simulink model "OptimizationCar"  (Simulink 8.8)
settings: Solver=FixedStepAuto  StartTime=0.0  StopTime=10.0  RelTol=1e-3
model workspace: external: MAT-File C:\Users\EMIdev1\Documents\GitHub\DRI001-MPS-2018.2.3-601-2\DRI006\DRIPSamples\CollisionWarningSystem\external\SlkModels\OptimizationCar.mat (data not in the file)
undefined symbols (not defined in the file or in its folder): detectionRange, driverReacionTime, frictionCoef, subjectPosition, subjectVelocity, targetPosition, targetVelocity
(part 1 of 2)
settings Model: Creator=EMIdev1  LastModifiedBy=EMIdev1
settings DataIOCC: LimitDataPoints=off  SaveFormat=Dataset  SignalLoggingSaveFormat=Dataset
settings OptimizationCC: LifeSpan=auto
settings DebuggingCC: UnderspecifiedInitializationDetection=Simplified  MergeDetectMultiDrivingBlocksExec=error  FcnCallInpInsideContextMsg=error  StateNameClashWarn=none  SFUnexpectedBacktrackingDiag=error  SFNoUnconditionalDefaultTransitionDiag=error  SFExecutionAtInitializationDiag=warning
settings HardwareCC: ProdLargestAtomicFloat=Float  ProdIntDivRoundTo=Zero  ProdEndianess=LittleEndian  ProdHWDeviceType=Intel->x86-32 (Windows32)
settings ModelReferenceCC: PropagateSignalLabelsOutOfModel=on
settings GRTTargetCC: TargetLangStandard=C99 (ISO)  GeneratePreprocessorConditionals=Use local settings  CombineOutputUpdateFcns=on  GRTInterface=off
settings ConfigComp: CovMetricSettings=dwe  CovHtmlReporting=off  CovSaveCumulativeToWorkspaceVar=off  CovSaveSingleToWorkspaceVar=off  CovExternalEMLEnable=on

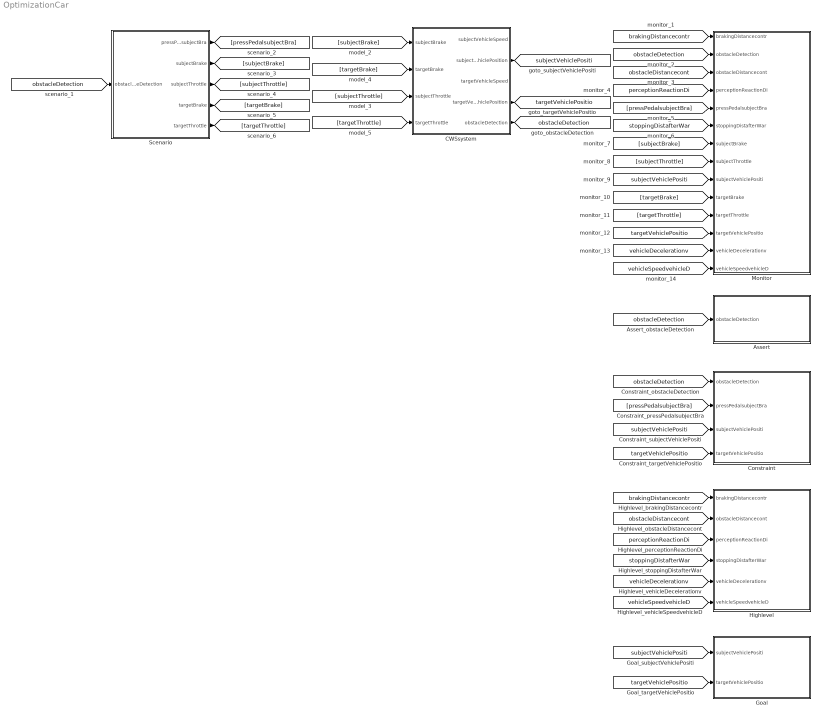
== system OptimizationCar ==
  Assert : Subsystem
  CWSsystem : Subsystem  LoadFcn=""
  Constraint : Subsystem
  Goal : Subsystem
  Highlevel : Subsystem
  Monitor : Subsystem
  Scenario : Subsystem
  tag scope: obstacleDetection=global, subjectVehiclePositi=global, targetVehiclePositio=global
  wires:
  [obstacleDetection] -> Scenario/1(obstacleDetection)
  Scenario/1(pressPedalsubjectBra) -> [pressPedalsubjectBra]
  Scenario/2(subjectBrake) -> [subjectBrake]
  [subjectBrake] -> CWSsystem/1(subjectBrake)
  Scenario/3(subjectThrottle) -> [subjectThrottle]
  [subjectThrottle] -> CWSsystem/3(subjectThrottle)
  Scenario/4(targetBrake) -> [targetBrake]
  [targetBrake] -> CWSsystem/2(targetBrake)
  Scenario/5(targetThrottle) -> [targetThrottle]
  [targetThrottle] -> CWSsystem/4(targetThrottle)
  [brakingDistancecontr] -> Monitor/1(brakingDistancecontr)
  [obstacleDetection] -> Monitor/2(obstacleDetection)
  [obstacleDistancecont] -> Monitor/3(obstacleDistancecont)
  [perceptionReactionDi] -> Monitor/4(perceptionReactionDi)
  [pressPedalsubjectBra] -> Monitor/5(pressPedalsubjectBra)
  [stoppingDistafterWar] -> Monitor/6(stoppingDistafterWar)
  [subjectBrake] -> Monitor/7(subjectBrake)
  [subjectThrottle] -> Monitor/8(subjectThrottle)
  [subjectVehiclePositi] -> Monitor/9(subjectVehiclePositi)
  [targetBrake] -> Monitor/10(targetBrake)
  [targetThrottle] -> Monitor/11(targetThrottle)
  [targetVehiclePositio] -> Monitor/12(targetVehiclePositio)
  [vehicleDecelerationv] -> Monitor/13(vehicleDecelerationv)
  [vehicleSpeedvehicleD] -> Monitor/14(vehicleSpeedvehicleD)
  [obstacleDetection] -> Assert/1(obstacleDetection)
  [obstacleDetection] -> Constraint/1(obstacleDetection)
  [pressPedalsubjectBra] -> Constraint/2(pressPedalsubjectBra)
  [subjectVehiclePositi] -> Constraint/3(subjectVehiclePositi)
  [targetVehiclePositio] -> Constraint/4(targetVehiclePositio)
  [brakingDistancecontr] -> Highlevel/1(brakingDistancecontr)
  [obstacleDistancecont] -> Highlevel/2(obstacleDistancecont)
  [perceptionReactionDi] -> Highlevel/3(perceptionReactionDi)
  [stoppingDistafterWar] -> Highlevel/4(stoppingDistafterWar)
  [vehicleDecelerationv] -> Highlevel/5(vehicleDecelerationv)
  [vehicleSpeedvehicleD] -> Highlevel/6(vehicleSpeedvehicleD)
  [subjectVehiclePositi] -> Goal/1(subjectVehiclePositi)
  [targetVehiclePositio] -> Goal/2(targetVehiclePositio)
  CWSsystem/5(obstacleDetection) -> [obstacleDetection]
  CWSsystem/2(subjectVehiclePosition) -> [subjectVehiclePositi]
  CWSsystem/4(targetVehiclePosition) -> [targetVehiclePositio]

== system OptimizationCar/Assert ==
  obstacleDetection : Inport
  Assert_1 : Subsystem
  simout_1 : ToFile  Filename=Assert_1.mat  MatrixName=Assert_1  SaveFormat=Timeseries
  wires:
  obstacleDetection/1 -> Assert_1/1(obstacleDetection)
  Assert_1/1(Assert_1) -> simout_1/1

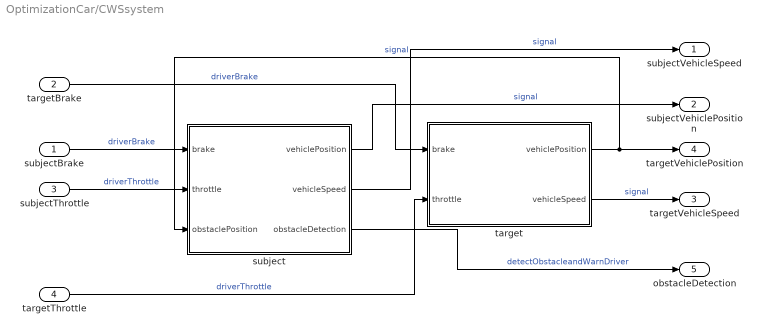
== system OptimizationCar/CWSsystem ==
  subjectBrake : Inport
      settings: AttributesFormatString=driverBrake
  targetBrake : Inport  Port=2
      settings: AttributesFormatString=driverBrake
  subjectThrottle : Inport  Port=3
      settings: AttributesFormatString=driverThrottle
  targetThrottle : Inport  Port=4
      settings: AttributesFormatString=driverThrottle
  subject : Subsystem  LoadFcn=""
  target : Subsystem  LoadFcn=""
  subjectVehicleSpeed : Outport
      settings: AttributesFormatString=signal
  subjectVehiclePosition : Outport  Port=2
      settings: AttributesFormatString=signal
  targetVehicleSpeed : Outport  Port=3
      settings: AttributesFormatString=signal
  targetVehiclePosition : Outport  Port=4
      settings: AttributesFormatString=signal
  obstacleDetection : Outport  Port=5
      settings: AttributesFormatString=detectObstacleandWarnDriver
  wires:
  subject/3(obstacleDetection) -> obstacleDetection/1  "detectObstacleandWarnDriver"
  target/2(vehicleSpeed) -> targetVehicleSpeed/1  "signal"
  subject/2(vehicleSpeed) -> subjectVehicleSpeed/1  "signal"
  subject/1(vehiclePosition) -> subjectVehiclePosition/1  "signal"
  targetThrottle/1 -> target/2(throttle)  "driverThrottle"
  subjectThrottle/1 -> subject/2(throttle)  "driverThrottle"
  targetBrake/1 -> target/1(brake)  "driverBrake"
  subjectBrake/1 -> subject/1(brake)  "driverBrake"
  target/1(vehiclePosition) -> targetVehiclePosition/1, subject/3(obstaclePosition)  "signal"

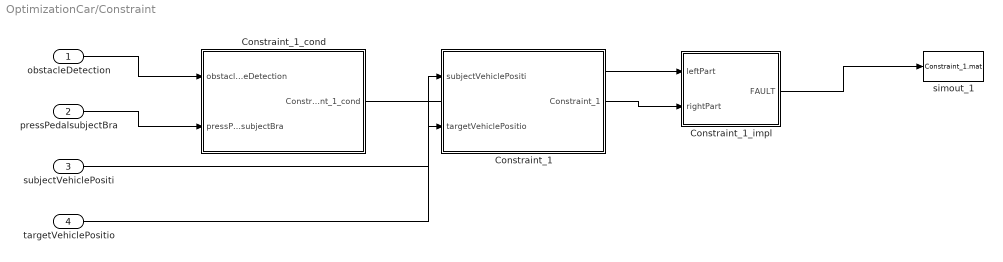
== system OptimizationCar/Constraint ==
  obstacleDetection : Inport
  pressPedalsubjectBra : Inport  Port=2
  subjectVehiclePositi : Inport  Port=3
  targetVehiclePositio : Inport  Port=4
  Constraint_1 : Subsystem
  Constraint_1_cond : Subsystem
  Constraint_1_impl : Subsystem  TreatAsAtomicUnit=on
  simout_1 : ToFile  Filename=Constraint_1.mat  MatrixName=Constraint_1  SaveFormat=Timeseries
  wires:
  obstacleDetection/1 -> Constraint_1_cond/1(obstacleDetection)
  pressPedalsubjectBra/1 -> Constraint_1_cond/2(pressPedalsubjectBra)
  Constraint_1_cond/1(Constraint_1_cond) -> Constraint_1_impl/1(leftPart)
  subjectVehiclePositi/1 -> Constraint_1/1(subjectVehiclePositi)
  targetVehiclePositio/1 -> Constraint_1/2(targetVehiclePositio)
  Constraint_1/1(Constraint_1) -> Constraint_1_impl/2(rightPart)
  Constraint_1_impl/1(FAULT) -> simout_1/1

== system OptimizationCar/Goal ==
  subjectVehiclePositi : Inport
  targetVehiclePositio : Inport  Port=2
  Goal_1 : Subsystem
  simout_1 : ToFile  Filename=Goal_1.mat  MatrixName=Goal_1  SaveFormat=Timeseries
  wires:
  subjectVehiclePositi/1 -> Goal_1/1(subjectVehiclePositi)
  targetVehiclePositio/1 -> Goal_1/2(targetVehiclePositio)
  Goal_1/1(Goal_1) -> simout_1/1

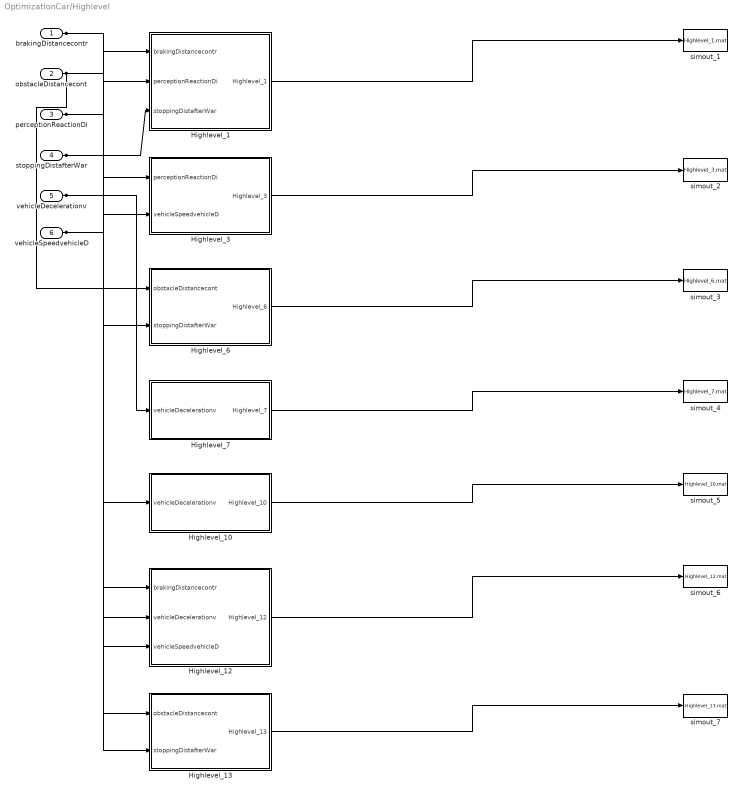
== system OptimizationCar/Highlevel ==
  brakingDistancecontr : Inport
  obstacleDistancecont : Inport  Port=2
  perceptionReactionDi : Inport  Port=3
  stoppingDistafterWar : Inport  Port=4
  vehicleDecelerationv : Inport  Port=5
  vehicleSpeedvehicleD : Inport  Port=6
  Highlevel_1 : Subsystem
  Highlevel_10 : Subsystem
  Highlevel_12 : Subsystem
  Highlevel_13 : Subsystem
  Highlevel_3 : Subsystem
  Highlevel_6 : Subsystem
  Highlevel_7 : Subsystem
  simout_1 : ToFile  Filename=Highlevel_1.mat  MatrixName=Highlevel_1  SaveFormat=Timeseries
  simout_2 : ToFile  Filename=Highlevel_3.mat  MatrixName=Highlevel_3  SaveFormat=Timeseries
  simout_3 : ToFile  Filename=Highlevel_6.mat  MatrixName=Highlevel_6  SaveFormat=Timeseries
  simout_4 : ToFile  Filename=Highlevel_7.mat  MatrixName=Highlevel_7  SaveFormat=Timeseries
  simout_5 : ToFile  Filename=Highlevel_10.mat  MatrixName=Highlevel_10  SaveFormat=Timeseries
  simout_6 : ToFile  Filename=Highlevel_12.mat  MatrixName=Highlevel_12  SaveFormat=Timeseries
  simout_7 : ToFile  Filename=Highlevel_13.mat  MatrixName=Highlevel_13  SaveFormat=Timeseries
  wires:
  brakingDistancecontr/1 -> Highlevel_1/1(brakingDistancecontr), Highlevel_12/1(brakingDistancecontr)
  perceptionReactionDi/1 -> Highlevel_1/2(perceptionReactionDi), Highlevel_3/1(perceptionReactionDi)
  stoppingDistafterWar/1 -> Highlevel_1/3(stoppingDistafterWar), Highlevel_6/2(stoppingDistafterWar), Highlevel_13/2(stoppingDistafterWar)
  Highlevel_1/1(Highlevel_1) -> simout_1/1
  vehicleSpeedvehicleD/1 -> Highlevel_3/2(vehicleSpeedvehicleD), Highlevel_12/3(vehicleSpeedvehicleD)
  Highlevel_3/1(Highlevel_3) -> simout_2/1
  obstacleDistancecont/1 -> Highlevel_6/1(obstacleDistancecont), Highlevel_13/1(obstacleDistancecont)
  Highlevel_6/1(Highlevel_6) -> simout_3/1
  vehicleDecelerationv/1 -> Highlevel_7/1(vehicleDecelerationv), Highlevel_10/1(vehicleDecelerationv), Highlevel_12/2(vehicleDecelerationv)
  Highlevel_7/1(Highlevel_7) -> simout_4/1
  Highlevel_10/1(Highlevel_10) -> simout_5/1
  Highlevel_12/1(Highlevel_12) -> simout_6/1
  Highlevel_13/1(Highlevel_13) -> simout_7/1

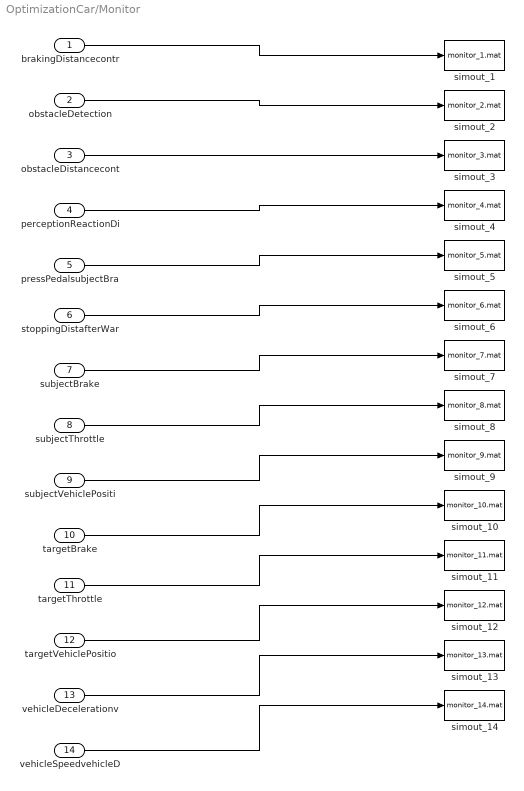
== system OptimizationCar/Monitor ==
  brakingDistancecontr : Inport
  obstacleDetection : Inport  Port=2
  obstacleDistancecont : Inport  Port=3
  perceptionReactionDi : Inport  Port=4
  pressPedalsubjectBra : Inport  Port=5
  stoppingDistafterWar : Inport  Port=6
  subjectBrake : Inport  Port=7
  subjectThrottle : Inport  Port=8
  subjectVehiclePositi : Inport  Port=9
  targetBrake : Inport  Port=10
  targetThrottle : Inport  Port=11
  targetVehiclePositio : Inport  Port=12
  vehicleDecelerationv : Inport  Port=13
  vehicleSpeedvehicleD : Inport  Port=14
  simout_1 : ToFile  Filename=monitor_1.mat  MatrixName=brakingDistancecontr  SaveFormat=Timeseries
  simout_10 : ToFile  Filename=monitor_10.mat  MatrixName=targetBrake  SaveFormat=Timeseries
  simout_11 : ToFile  Filename=monitor_11.mat  MatrixName=targetThrottle  SaveFormat=Timeseries
  simout_12 : ToFile  Filename=monitor_12.mat  MatrixName=targetVehiclePositio  SaveFormat=Timeseries
  simout_13 : ToFile  Filename=monitor_13.mat  MatrixName=vehicleDecelerationv  SaveFormat=Timeseries
  simout_14 : ToFile  Filename=monitor_14.mat  MatrixName=vehicleSpeedvehicleD  SaveFormat=Timeseries
  simout_2 : ToFile  Filename=monitor_2.mat  MatrixName=obstacleDetection  SaveFormat=Timeseries
  simout_3 : ToFile  Filename=monitor_3.mat  MatrixName=obstacleDistancecont  SaveFormat=Timeseries
  simout_4 : ToFile  Filename=monitor_4.mat  MatrixName=perceptionReactionDi  SaveFormat=Timeseries
  simout_5 : ToFile  Filename=monitor_5.mat  MatrixName=pressPedalsubjectBra  SaveFormat=Timeseries
  simout_6 : ToFile  Filename=monitor_6.mat  MatrixName=stoppingDistafterWar  SaveFormat=Timeseries
  simout_7 : ToFile  Filename=monitor_7.mat  MatrixName=subjectBrake  SaveFormat=Timeseries
  simout_8 : ToFile  Filename=monitor_8.mat  MatrixName=subjectThrottle  SaveFormat=Timeseries
  simout_9 : ToFile  Filename=monitor_9.mat  MatrixName=subjectVehiclePositi  SaveFormat=Timeseries
  wires:
  brakingDistancecontr/1 -> simout_1/1
  obstacleDetection/1 -> simout_2/1
  obstacleDistancecont/1 -> simout_3/1
  perceptionReactionDi/1 -> simout_4/1
  pressPedalsubjectBra/1 -> simout_5/1
  stoppingDistafterWar/1 -> simout_6/1
  subjectBrake/1 -> simout_7/1
  subjectThrottle/1 -> simout_8/1
  subjectVehiclePositi/1 -> simout_9/1
  targetBrake/1 -> simout_10/1
  targetThrottle/1 -> simout_11/1
  targetVehiclePositio/1 -> simout_12/1
  vehicleDecelerationv/1 -> simout_13/1
  vehicleSpeedvehicleD/1 -> simout_14/1

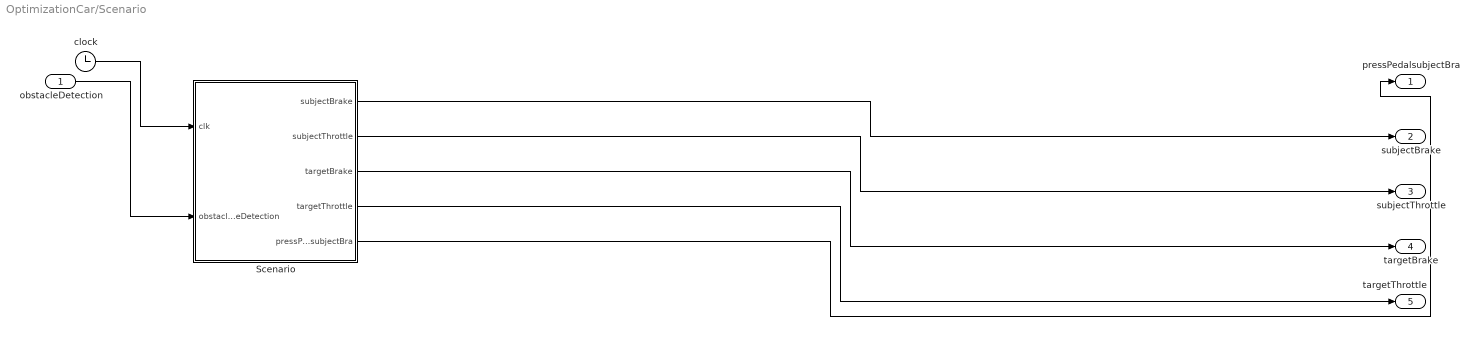
== system OptimizationCar/Scenario ==
  obstacleDetection : Inport
  Scenario : Stateflow chart  TreatAsAtomicUnit=on
  clock : Clock
  pressPedalsubjectBra : Outport
  subjectBrake : Outport  Port=2
  subjectThrottle : Outport  Port=3
  targetBrake : Outport  Port=4
  targetThrottle : Outport  Port=5
  wires:
  clock/1 -> Scenario/1(clk)
  obstacleDetection/1 -> Scenario/2(obstacleDetection)
  Scenario/1(subjectBrake) -> subjectBrake/1
  Scenario/2(subjectThrottle) -> subjectThrottle/1
  Scenario/3(targetBrake) -> targetBrake/1
  Scenario/4(targetThrottle) -> targetThrottle/1
  Scenario/5(pressPedalsubjectBra) -> pressPedalsubjectBra/1

== system OptimizationCar/Assert/Assert_1 ==
  obstacleDetection : Inport
  existsAndStay : Subsystem  TreatAsAtomicUnit=on
  globally : Subsystem  TreatAsAtomicUnit=on
  Assert_1 : Outport
  wires:
  globally/1(qualifierTrue) -> existsAndStay/2(Enable)
  obstacleDetection/1 -> existsAndStay/1(instTrue)
  existsAndStay/1(FAULT) -> Assert_1/1

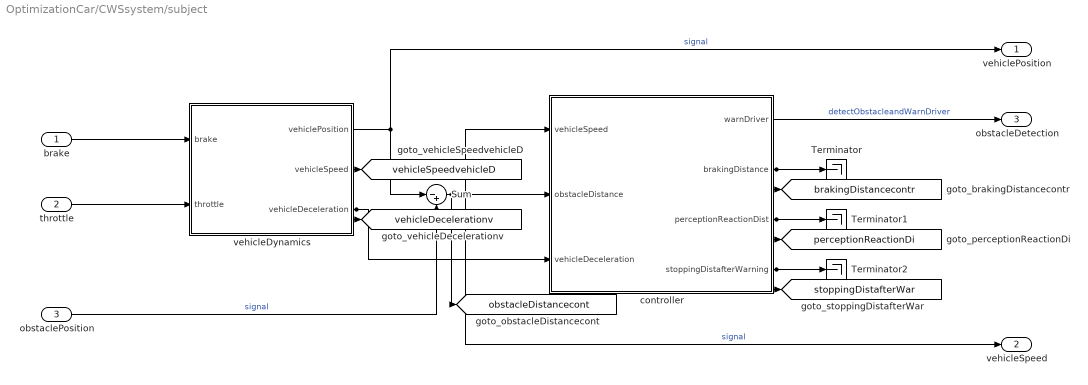
== system OptimizationCar/CWSsystem/subject ==
  brake : Inport
  throttle : Inport  Port=2
  obstaclePosition : Inport  Port=3
      settings: AttributesFormatString=signal
  Sum : Sum  Inputs=|-+
  Terminator : Terminator
  Terminator1 : Terminator
  Terminator2 : Terminator
  controller : Subsystem
      settings: AttributesFormatString=CWS
  vehicleDynamics : Subsystem
  vehiclePosition : Outport
      settings: AttributesFormatString=signal
  vehicleSpeed : Outport  Port=2
      settings: AttributesFormatString=signal
  obstacleDetection : Outport  Port=3
      settings: AttributesFormatString=signal
  tag scope: brakingDistancecontr=global, obstacleDistancecont=global, perceptionReactionDi=global, stoppingDistafterWar=global, vehicleDecelerationv=global, vehicleSpeedvehicleD=global
  wires:
  controller/4(stoppingDistafterWarning) -> Terminator2/1, [stoppingDistafterWar]
  controller/3(perceptionReactionDist) -> Terminator1/1, [perceptionReactionDi]
  vehicleDynamics/3(vehicleDeceleration) -> controller/3(vehicleDeceleration), [vehicleDecelerationv]
  controller/2(brakingDistance) -> Terminator/1, [brakingDistancecontr]
  obstaclePosition/1 -> Sum/2  "signal"
  Sum/1 -> controller/2(obstacleDistance), [obstacleDistancecont]
  brake/1 -> vehicleDynamics/1(brake)
  throttle/1 -> vehicleDynamics/2(throttle)
  controller/1(warnDriver) -> obstacleDetection/1  "detectObstacleandWarnDriver"
  vehicleDynamics/2(vehicleSpeed) -> vehicleSpeed/1, controller/1(vehicleSpeed), [vehicleSpeedvehicleD]  "signal"
  vehicleDynamics/1(vehiclePosition) -> vehiclePosition/1, Sum/1  "signal"

== system OptimizationCar/CWSsystem/target ==
  brake : Inport
  throttle : Inport  Port=2
  vehicleDynamics : Subsystem  Variant=on  OverrideUsingVariant=truck
  vehiclePosition : Outport
      settings: AttributesFormatString=signal
  vehicleSpeed : Outport  Port=2
      settings: AttributesFormatString=signal
  wires:
  brake/1 -> vehicleDynamics/1(brake)
  throttle/1 -> vehicleDynamics/2(throttle)
  vehicleDynamics/2(vehicleSpeed) -> vehicleSpeed/1  "signal"
  vehicleDynamics/1(vehiclePosition) -> vehiclePosition/1  "signal"

== system OptimizationCar/Constraint/Constraint_1 ==
  subjectVehiclePositi : Inport
  targetVehiclePositio : Inport  Port=2
  LessExpression_3_4 : RelationalOperator  Operator=<  OutDataTypeStr=boolean  RndMeth=Simplest
  MinusExpression_2_4 : Sum  Inputs=+-
  NumberLiteral_1_4 : Constant  Value=2
  globally : Subsystem  TreatAsAtomicUnit=on
  universally : Subsystem  TreatAsAtomicUnit=on
  Constraint_1 : Outport
  wires:
  targetVehiclePositio/1 -> MinusExpression_2_4/1
  NumberLiteral_1_4/1 -> MinusExpression_2_4/2
  subjectVehiclePositi/1 -> LessExpression_3_4/1
  MinusExpression_2_4/1 -> LessExpression_3_4/2
  globally/1(qualifierTrue) -> universally/Enable
  LessExpression_3_4/1 -> universally/1(instTrue)
  universally/1(FAULT) -> Constraint_1/1

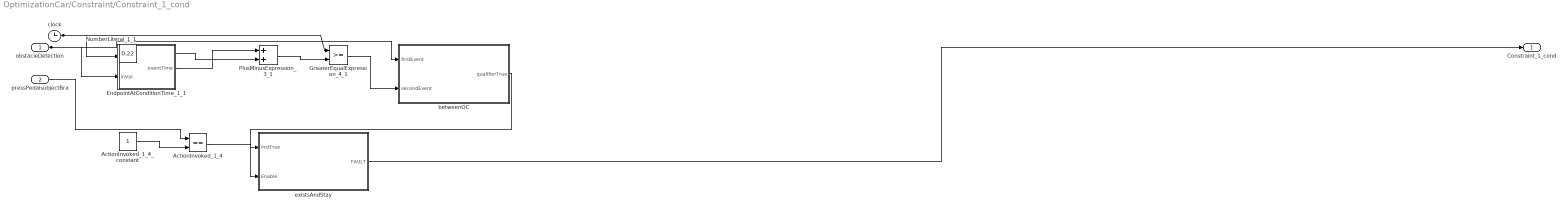
== system OptimizationCar/Constraint/Constraint_1_cond ==
  obstacleDetection : Inport
  pressPedalsubjectBra : Inport  Port=2
  ActionInvoked_1_4 : RelationalOperator  Operator===  OutDataTypeStr=boolean  RndMeth=Simplest
  ActionInvoked_1_4_constant : Constant
  EndpointAtConditionTime_1_1 : Subsystem
  GreaterEqualExpression_4_1 : RelationalOperator  OutDataTypeStr=boolean  RndMeth=Simplest
  NumberLiteral_1_1 : Constant  Value=0.22
  PlusMinusExpression_3_1 : Sum
  betweenOC : Subsystem  TreatAsAtomicUnit=on
  clock : Clock
  existsAndStay : Subsystem  TreatAsAtomicUnit=on
  Constraint_1_cond : Outport
  wires:
  clock/1 -> EndpointAtConditionTime_1_1/1(clk), GreaterEqualExpression_4_1/1
  obstacleDetection/1 -> EndpointAtConditionTime_1_1/2(inVal), betweenOC/1(firstEvent)
  EndpointAtConditionTime_1_1/1(eventTime) -> PlusMinusExpression_3_1/1
  NumberLiteral_1_1/1 -> PlusMinusExpression_3_1/2
  PlusMinusExpression_3_1/1 -> GreaterEqualExpression_4_1/2
  GreaterEqualExpression_4_1/1 -> betweenOC/2(secondEvent)
  pressPedalsubjectBra/1 -> ActionInvoked_1_4/1
  ActionInvoked_1_4_constant/1 -> ActionInvoked_1_4/2
  betweenOC/1(qualifierTrue) -> existsAndStay/2(Enable)
  ActionInvoked_1_4/1 -> existsAndStay/1(instTrue)
  existsAndStay/1(FAULT) -> Constraint_1_cond/1

== system OptimizationCar/Constraint/Constraint_1_impl ==
  leftPart : Inport
  rightPart : Inport  Port=2
  Implication : Subsystem
  Logical Operator : Logic  Operator=NOT  AllPortsSameDT=off  OutDataTypeStr=boolean
  Logical Operator1 : Logic  Operator=NOT  AllPortsSameDT=off  OutDataTypeStr=boolean
  Logical Operator2 : Logic  Operator=NOT  AllPortsSameDT=off  OutDataTypeStr=boolean
  FAULT : Outport  InitialOutput=0
  wires:
  Logical Operator2/1 -> FAULT/1
  Implication/1(Out1) -> Logical Operator2/1
  Logical Operator1/1 -> Implication/1(In1)
  Logical Operator/1 -> Implication/Enable
  rightPart/1 -> Logical Operator1/1
  leftPart/1 -> Logical Operator/1

== system OptimizationCar/Goal/Goal_1 ==
  subjectVehiclePositi : Inport
  targetVehiclePositio : Inport  Port=2
  MinusExpression_1_1 : Sum  Inputs=+-
  UnaryMinusExpression_1_1 : UnaryMinus
  Goal_1 : Outport
  wires:
  targetVehiclePositio/1 -> MinusExpression_1_1/1
  subjectVehiclePositi/1 -> MinusExpression_1_1/2
  MinusExpression_1_1/1 -> UnaryMinusExpression_1_1/1
  UnaryMinusExpression_1_1/1 -> Goal_1/1

== system OptimizationCar/Highlevel/Highlevel_1 ==
  brakingDistancecontr : Inport
  perceptionReactionDi : Inport  Port=2
  stoppingDistafterWar : Inport  Port=3
  AssignmentExpr_2_4 : RelationalOperator  Operator===  OutDataTypeStr=boolean  RndMeth=Simplest
  PlusExpression_1_4 : Sum
  globally : Subsystem  TreatAsAtomicUnit=on
  universally : Subsystem  TreatAsAtomicUnit=on
  Highlevel_1 : Outport
  wires:
  perceptionReactionDi/1 -> PlusExpression_1_4/1
  brakingDistancecontr/1 -> PlusExpression_1_4/2
  stoppingDistafterWar/1 -> AssignmentExpr_2_4/1
  PlusExpression_1_4/1 -> AssignmentExpr_2_4/2
  globally/1(qualifierTrue) -> universally/Enable
  AssignmentExpr_2_4/1 -> universally/1(instTrue)
  universally/1(FAULT) -> Highlevel_1/1

== system OptimizationCar/Highlevel/Highlevel_10 ==
  vehicleDecelerationv : Inport
  LessExpression_3_4 : RelationalOperator  Operator=<  OutDataTypeStr=boolean  RndMeth=Simplest
  MultiExpression_2_4 : Product  Inputs=**
  NumberLiteral_1_5 : Constant  Value=9.8
  SimulinkReference_1_4 : Constant  Value=frictionCoef
  globally : Subsystem  TreatAsAtomicUnit=on
  universally : Subsystem  TreatAsAtomicUnit=on
  Highlevel_10 : Outport
  wires:
  SimulinkReference_1_4/1 -> MultiExpression_2_4/1
  NumberLiteral_1_5/1 -> MultiExpression_2_4/2
  vehicleDecelerationv/1 -> LessExpression_3_4/1
  MultiExpression_2_4/1 -> LessExpression_3_4/2
  globally/1(qualifierTrue) -> universally/Enable
  LessExpression_3_4/1 -> universally/1(instTrue)
  universally/1(FAULT) -> Highlevel_10/1

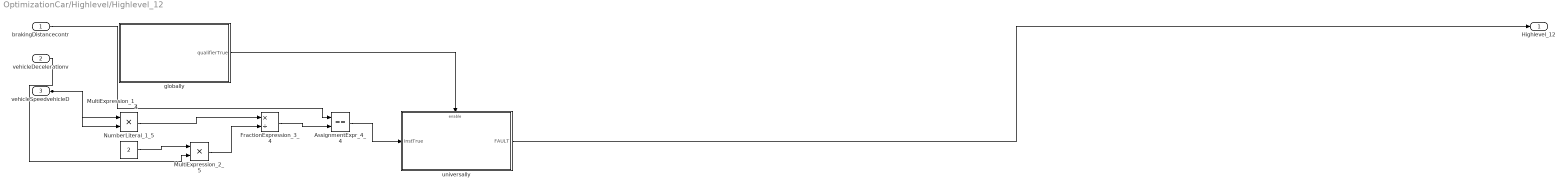
== system OptimizationCar/Highlevel/Highlevel_12 ==
  brakingDistancecontr : Inport
  vehicleDecelerationv : Inport  Port=2
  vehicleSpeedvehicleD : Inport  Port=3
  AssignmentExpr_4_4 : RelationalOperator  Operator===  OutDataTypeStr=boolean  RndMeth=Simplest
  FractionExpression_3_4 : Product  Inputs=*/
  MultiExpression_1_4 : Product  Inputs=**
  MultiExpression_2_5 : Product  Inputs=**
  NumberLiteral_1_5 : Constant  Value=2
  globally : Subsystem  TreatAsAtomicUnit=on
  universally : Subsystem  TreatAsAtomicUnit=on
  Highlevel_12 : Outport
  wires:
  vehicleSpeedvehicleD/1 -> MultiExpression_1_4/1, MultiExpression_1_4/2
  NumberLiteral_1_5/1 -> MultiExpression_2_5/1
  vehicleDecelerationv/1 -> MultiExpression_2_5/2
  MultiExpression_1_4/1 -> FractionExpression_3_4/1
  MultiExpression_2_5/1 -> FractionExpression_3_4/2
  brakingDistancecontr/1 -> AssignmentExpr_4_4/1
  FractionExpression_3_4/1 -> AssignmentExpr_4_4/2
  globally/1(qualifierTrue) -> universally/Enable
  AssignmentExpr_4_4/1 -> universally/1(instTrue)
  universally/1(FAULT) -> Highlevel_12/1

== system OptimizationCar/Highlevel/Highlevel_13 ==
  obstacleDistancecont : Inport
  stoppingDistafterWar : Inport  Port=2
  GreaterExpression_2_4 : RelationalOperator  Operator=>  OutDataTypeStr=boolean  RndMeth=Simplest
  MinusExpression_1_4 : Sum  Inputs=+-
  NumberLiteral_1_5 : Constant  Value=3
  globally : Subsystem  TreatAsAtomicUnit=on
  universally : Subsystem  TreatAsAtomicUnit=on
  Highlevel_13 : Outport
  wires:
  obstacleDistancecont/1 -> MinusExpression_1_4/1
  stoppingDistafterWar/1 -> MinusExpression_1_4/2
  MinusExpression_1_4/1 -> GreaterExpression_2_4/1
  NumberLiteral_1_5/1 -> GreaterExpression_2_4/2
  globally/1(qualifierTrue) -> universally/Enable
  GreaterExpression_2_4/1 -> universally/1(instTrue)
  universally/1(FAULT) -> Highlevel_13/1

== system OptimizationCar/Highlevel/Highlevel_3 ==
  perceptionReactionDi : Inport
  vehicleSpeedvehicleD : Inport  Port=2
  AssignmentExpr_3_4 : RelationalOperator  Operator===  OutDataTypeStr=boolean  RndMeth=Simplest
  MultiExpression_2_4 : Product  Inputs=**
  SimulinkReference_1_4 : Constant  Value=driverReacionTime
  globally : Subsystem  TreatAsAtomicUnit=on
  universally : Subsystem  TreatAsAtomicUnit=on
  Highlevel_3 : Outport
  wires:
  vehicleSpeedvehicleD/1 -> MultiExpression_2_4/1
  SimulinkReference_1_4/1 -> MultiExpression_2_4/2
  perceptionReactionDi/1 -> AssignmentExpr_3_4/1
  MultiExpression_2_4/1 -> AssignmentExpr_3_4/2
  globally/1(qualifierTrue) -> universally/Enable
  AssignmentExpr_3_4/1 -> universally/1(instTrue)
  universally/1(FAULT) -> Highlevel_3/1

== system OptimizationCar/Highlevel/Highlevel_6 ==
  obstacleDistancecont : Inport
  stoppingDistafterWar : Inport  Port=2
  LessExpression_1_4 : RelationalOperator  Operator=<  OutDataTypeStr=boolean  RndMeth=Simplest
  globally : Subsystem  TreatAsAtomicUnit=on
  universally : Subsystem  TreatAsAtomicUnit=on
  Highlevel_6 : Outport
  wires:
  stoppingDistafterWar/1 -> LessExpression_1_4/1
  obstacleDistancecont/1 -> LessExpression_1_4/2
  globally/1(qualifierTrue) -> universally/Enable
  LessExpression_1_4/1 -> universally/1(instTrue)
  universally/1(FAULT) -> Highlevel_6/1

== system OptimizationCar/Highlevel/Highlevel_7 ==
  vehicleDecelerationv : Inport
  LessExpression_2_4 : RelationalOperator  Operator=<  OutDataTypeStr=boolean  RndMeth=Simplest
  NumberLiteral_1_4 : Constant  Value=4.9
  globally : Subsystem  TreatAsAtomicUnit=on
  universally : Subsystem  TreatAsAtomicUnit=on
  Highlevel_7 : Outport
  wires:
  vehicleDecelerationv/1 -> LessExpression_2_4/1
  NumberLiteral_1_4/1 -> LessExpression_2_4/2
  globally/1(qualifierTrue) -> universally/Enable
  LessExpression_2_4/1 -> universally/1(instTrue)
  universally/1(FAULT) -> Highlevel_7/1

== system OptimizationCar/Assert/Assert_1/existsAndStay ==
  instTrue : Inport
  Enable : Inport  Port=2
  Logical Operator : Logic  Operator=OR  AllPortsSameDT=off  OutDataTypeStr=boolean
  Logical Operator2 : Logic  Operator=NOT  AllPortsSameDT=off  OutDataTypeStr=boolean
  Triggered Subsystem : Subsystem  TreatAsAtomicUnit=on
  last : Subsystem  TreatAsAtomicUnit=on
  universally : Subsystem  TreatAsAtomicUnit=on
  FAULT : Outport  InitialOutput=0
  wires:
  Logical Operator2/1 -> Logical Operator/1
  Triggered Subsystem/1(Out1) -> universally/Enable
  universally/1(FAULT) -> Logical Operator/2
  Enable/1 -> Triggered Subsystem/Trigger, last/Enable
  last/1(TRUE) -> Logical Operator2/1
  Logical Operator/1 -> FAULT/1
  instTrue/1 -> last/1(instTrue), universally/1(instTrue)

== system OptimizationCar/Assert/Assert_1/globally ==
  Constant : Constant  OutDataTypeStr=boolean
  qualifierTrue : Outport
  wires:
  Constant/1 -> qualifierTrue/1

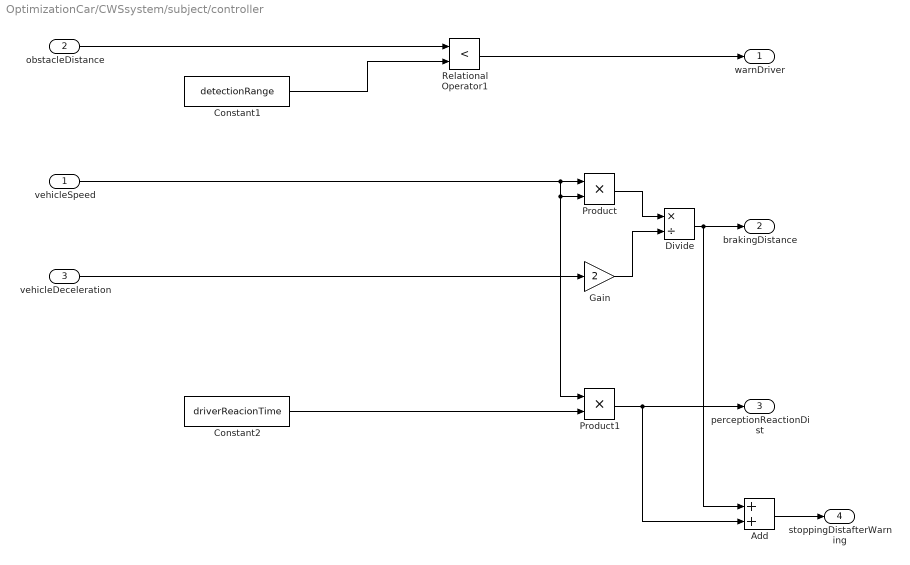
== system OptimizationCar/CWSsystem/subject/controller ==
  vehicleSpeed : Inport
      settings: AttributesFormatString=signal
  obstacleDistance : Inport  Port=2
      settings: AttributesFormatString=signal
  vehicleDeceleration : Inport  Port=3
      settings: AttributesFormatString=signal
  Add : Sum
  Constant1 : Constant  Value=detectionRange
  Constant2 : Constant  Value=driverReacionTime
  Divide : Product  Inputs=*/
  Gain : Gain  Gain=2
  Product : Product
  Product1 : Product
  Relational Operator1 : RelationalOperator  Operator=<  OutDataTypeStr=boolean  RndMeth=Nearest
  warnDriver : Outport
      settings: AttributesFormatString=detectObstacleandWarnDriver
  brakingDistance : Outport  Port=2
  perceptionReactionDist : Outport  Port=3
  stoppingDistafterWarning : Outport  Port=4
  wires:
  Constant1/1 -> Relational Operator1/2
  Add/1 -> stoppingDistafterWarning/1
  Constant2/1 -> Product1/2
  Product1/1 -> perceptionReactionDist/1, Add/2
  Divide/1 -> brakingDistance/1, Add/1
  vehicleSpeed/1 -> Product1/1, Product/2, Product/1
  Product/1 -> Divide/1
  Gain/1 -> Divide/2
  vehicleDeceleration/1 -> Gain/1
  Relational Operator1/1 -> warnDriver/1
  obstacleDistance/1 -> Relational Operator1/1

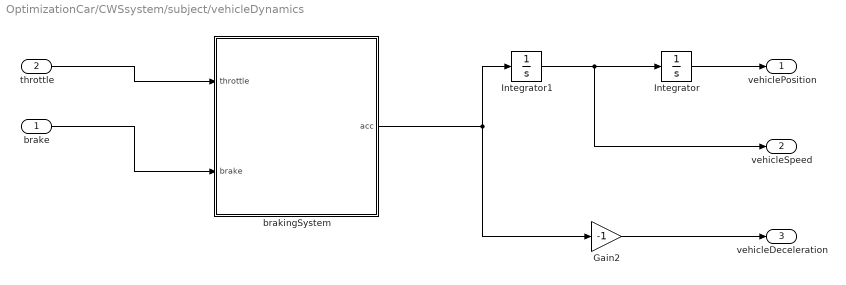
== system OptimizationCar/CWSsystem/subject/vehicleDynamics ==
  brake : Inport
  throttle : Inport  Port=2
  Gain2 : Gain  Gain=-1
  Integrator : Integrator  InitialCondition=subjectPosition
  Integrator1 : Integrator  InitialCondition=subjectVelocity  LimitOutput=on  LowerSaturationLimit=0
  brakingSystem : Subsystem
  vehiclePosition : Outport
      settings: AttributesFormatString=signal
  vehicleSpeed : Outport  Port=2
      settings: AttributesFormatString=signal
  vehicleDeceleration : Outport  Port=3
      settings: AttributesFormatString=signal
  wires:
  brake/1 -> brakingSystem/2(brake)
  throttle/1 -> brakingSystem/1(throttle)
  brakingSystem/1(acc) -> Gain2/1, Integrator1/1
  Gain2/1 -> vehicleDeceleration/1
  Integrator1/1 -> Integrator/1, vehicleSpeed/1
  Integrator/1 -> vehiclePosition/1

== system OptimizationCar/CWSsystem/target/vehicleDynamics ==
  note: 1) Add Subsystem or Model blocks as valid variant choices.
      | 2) You cannot connect blocks at this level. At simulation, connectivity is automatically
      | determined, based on the active variant and port name matching.
  brake : Inport
  throttle : Inport  Port=2
  car : Subsystem  VariantControl=car
  truck : Subsystem  VariantControl=truck
  vehiclePosition : Outport
  vehicleSpeed : Outport  Port=2

== system OptimizationCar/Constraint/Constraint_1/globally ==
  Constant : Constant  OutDataTypeStr=boolean
  qualifierTrue : Outport
  wires:
  Constant/1 -> qualifierTrue/1

== system OptimizationCar/Constraint/Constraint_1/universally ==
  instTrue : Inport
  Enable : EnablePort
  Logical Operator1 : Logic  Operator=NOT  AllPortsSameDT=off  OutDataTypeStr=boolean
  from : Subsystem  TreatAsAtomicUnit=on
  FAULT : Outport  InitialOutput=0
  wires:
  Logical Operator1/1 -> from/1(instTrue)
  instTrue/1 -> Logical Operator1/1
  from/1(qualifierTrue) -> FAULT/1

== system OptimizationCar/Constraint/Constraint_1_cond/EndpointAtConditionTime_1_1 ==
  clk : Inport
  inVal : Inport  Port=2
  Constant : Constant  Value=Inf
  Terminator : Terminator
  Terminator1 : Terminator
  detectEventTime : Stateflow chart  TreatAsAtomicUnit=on
  eventTime : Outport
  wires:
  Constant/1 -> detectEventTime/3(init)
  detectEventTime/3(isTrue) -> Terminator1/1
  detectEventTime/1(elapsedTime) -> Terminator/1
  detectEventTime/2(eventTime) -> eventTime/1
  inVal/1 -> detectEventTime/2(inVal)
  clk/1 -> detectEventTime/1(clk)

== system OptimizationCar/Constraint/Constraint_1_cond/betweenOC ==
  firstEvent : Inport
  secondEvent : Inport  Port=2
  Logical Operator : Logic  AllPortsSameDT=off  OutDataTypeStr=boolean
  after : Subsystem  TreatAsAtomicUnit=on
  until : Subsystem  TreatAsAtomicUnit=on
  qualifierTrue : Outport
  wires:
  until/1(qualifierTrue) -> Logical Operator/2
  after/1(qualifierTrue) -> Logical Operator/1
  Logical Operator/1 -> qualifierTrue/1
  firstEvent/1 -> after/1(instTrue)
  secondEvent/1 -> until/1(instTrue)

== system OptimizationCar/Constraint/Constraint_1_cond/existsAndStay ==
  instTrue : Inport
  Enable : Inport  Port=2
  Logical Operator : Logic  Operator=OR  AllPortsSameDT=off  OutDataTypeStr=boolean
  Logical Operator2 : Logic  Operator=NOT  AllPortsSameDT=off  OutDataTypeStr=boolean
  Triggered Subsystem : Subsystem  TreatAsAtomicUnit=on
  last : Subsystem  TreatAsAtomicUnit=on
  universally : Subsystem  TreatAsAtomicUnit=on
  FAULT : Outport  InitialOutput=0
  wires:
  Logical Operator2/1 -> Logical Operator/1
  Triggered Subsystem/1(Out1) -> universally/Enable
  universally/1(FAULT) -> Logical Operator/2
  Enable/1 -> Triggered Subsystem/Trigger, last/Enable
  last/1(TRUE) -> Logical Operator2/1
  Logical Operator/1 -> FAULT/1
  instTrue/1 -> last/1(instTrue), universally/1(instTrue)

== system OptimizationCar/Constraint/Constraint_1_impl/Implication ==
  In1 : Inport
  Enable : EnablePort
  Out1 : Outport  OutputWhenDisabled=reset  InitialOutput=1
  wires:
  In1/1 -> Out1/1

== system OptimizationCar/Highlevel/Highlevel_1/globally ==
  Constant : Constant  OutDataTypeStr=boolean
  qualifierTrue : Outport
  wires:
  Constant/1 -> qualifierTrue/1

== system OptimizationCar/Highlevel/Highlevel_1/universally ==
  instTrue : Inport
  Enable : EnablePort
  Logical Operator1 : Logic  Operator=NOT  AllPortsSameDT=off  OutDataTypeStr=boolean
  from : Subsystem  TreatAsAtomicUnit=on
  FAULT : Outport  InitialOutput=0
  wires:
  Logical Operator1/1 -> from/1(instTrue)
  instTrue/1 -> Logical Operator1/1
  from/1(qualifierTrue) -> FAULT/1

== system OptimizationCar/Highlevel/Highlevel_10/globally ==
  Constant : Constant  OutDataTypeStr=boolean
  qualifierTrue : Outport
  wires:
  Constant/1 -> qualifierTrue/1

== system OptimizationCar/Highlevel/Highlevel_10/universally ==
  instTrue : Inport
  Enable : EnablePort
  Logical Operator1 : Logic  Operator=NOT  AllPortsSameDT=off  OutDataTypeStr=boolean
  from : Subsystem  TreatAsAtomicUnit=on
  FAULT : Outport  InitialOutput=0
  wires:
  Logical Operator1/1 -> from/1(instTrue)
  instTrue/1 -> Logical Operator1/1
  from/1(qualifierTrue) -> FAULT/1

== system OptimizationCar/Highlevel/Highlevel_12/globally ==
  Constant : Constant  OutDataTypeStr=boolean
  qualifierTrue : Outport
  wires:
  Constant/1 -> qualifierTrue/1

== system OptimizationCar/Highlevel/Highlevel_12/universally ==
  instTrue : Inport
  Enable : EnablePort
  Logical Operator1 : Logic  Operator=NOT  AllPortsSameDT=off  OutDataTypeStr=boolean
  from : Subsystem  TreatAsAtomicUnit=on
  FAULT : Outport  InitialOutput=0
  wires:
  Logical Operator1/1 -> from/1(instTrue)
  instTrue/1 -> Logical Operator1/1
  from/1(qualifierTrue) -> FAULT/1

== system OptimizationCar/Highlevel/Highlevel_13/globally ==
  Constant : Constant  OutDataTypeStr=boolean
  qualifierTrue : Outport
  wires:
  Constant/1 -> qualifierTrue/1

== system OptimizationCar/Highlevel/Highlevel_13/universally ==
  instTrue : Inport
  Enable : EnablePort
  Logical Operator1 : Logic  Operator=NOT  AllPortsSameDT=off  OutDataTypeStr=boolean
  from : Subsystem  TreatAsAtomicUnit=on
  FAULT : Outport  InitialOutput=0
  wires:
  Logical Operator1/1 -> from/1(instTrue)
  instTrue/1 -> Logical Operator1/1
  from/1(qualifierTrue) -> FAULT/1

== system OptimizationCar/Highlevel/Highlevel_3/globally ==
  Constant : Constant  OutDataTypeStr=boolean
  qualifierTrue : Outport
  wires:
  Constant/1 -> qualifierTrue/1

== system OptimizationCar/Highlevel/Highlevel_3/universally ==
  instTrue : Inport
  Enable : EnablePort
  Logical Operator1 : Logic  Operator=NOT  AllPortsSameDT=off  OutDataTypeStr=boolean
  from : Subsystem  TreatAsAtomicUnit=on
  FAULT : Outport  InitialOutput=0
  wires:
  Logical Operator1/1 -> from/1(instTrue)
  instTrue/1 -> Logical Operator1/1
  from/1(qualifierTrue) -> FAULT/1

== system OptimizationCar/Highlevel/Highlevel_6/globally ==
  Constant : Constant  OutDataTypeStr=boolean
  qualifierTrue : Outport
  wires:
  Constant/1 -> qualifierTrue/1

== system OptimizationCar/Highlevel/Highlevel_6/universally ==
  instTrue : Inport
  Enable : EnablePort
  Logical Operator1 : Logic  Operator=NOT  AllPortsSameDT=off  OutDataTypeStr=boolean
  from : Subsystem  TreatAsAtomicUnit=on
  FAULT : Outport  InitialOutput=0
  wires:
  Logical Operator1/1 -> from/1(instTrue)
  instTrue/1 -> Logical Operator1/1
  from/1(qualifierTrue) -> FAULT/1

== system OptimizationCar/Highlevel/Highlevel_7/globally ==
  Constant : Constant  OutDataTypeStr=boolean
  qualifierTrue : Outport
  wires:
  Constant/1 -> qualifierTrue/1

== system OptimizationCar/Highlevel/Highlevel_7/universally ==
  instTrue : Inport
  Enable : EnablePort
  Logical Operator1 : Logic  Operator=NOT  AllPortsSameDT=off  OutDataTypeStr=boolean
  from : Subsystem  TreatAsAtomicUnit=on
  FAULT : Outport  InitialOutput=0
  wires:
  Logical Operator1/1 -> from/1(instTrue)
  instTrue/1 -> Logical Operator1/1
  from/1(qualifierTrue) -> FAULT/1

== system OptimizationCar/Assert/Assert_1/existsAndStay/Triggered Subsystem ==
  Trigger : TriggerPort  TriggerType=falling  VariantControl=Variant
  Constant : Constant
  Out1 : Outport  InitialOutput=0
  wires:
  Constant/1 -> Out1/1

== system OptimizationCar/Assert/Assert_1/existsAndStay/last ==
  instTrue : Inport
  Enable : EnablePort
  TRUE : Outport  InitialOutput=1
  wires:
  instTrue/1 -> TRUE/1

== system OptimizationCar/Assert/Assert_1/existsAndStay/universally ==
  instTrue : Inport
  Enable : EnablePort
  Logical Operator1 : Logic  Operator=NOT  AllPortsSameDT=off  OutDataTypeStr=boolean
  from : Subsystem  TreatAsAtomicUnit=on
  FAULT : Outport  InitialOutput=0
  wires:
  from/1(qualifierTrue) -> FAULT/1
  instTrue/1 -> Logical Operator1/1
  Logical Operator1/1 -> from/1(instTrue)

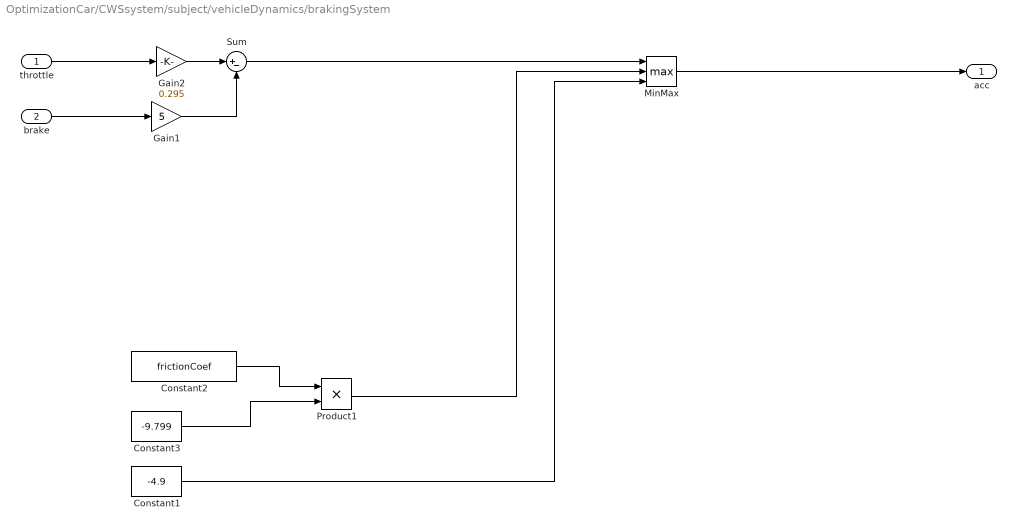
== system OptimizationCar/CWSsystem/subject/vehicleDynamics/brakingSystem ==
  throttle : Inport
  brake : Inport  Port=2
  Constant1 : Constant  Value=-4.9
  Constant2 : Constant  Value=frictionCoef
  Constant3 : Constant  Value=-9.799
  Gain1 : Gain  Gain=5
  Gain2 : Gain  Gain=0.295
  MinMax : MinMax  Function=max  Inputs=3
  Product1 : Product
  Sum : Sum  Inputs=|+-
  acc : Outport
  wires:
  Gain2/1 -> Sum/1
  Gain1/1 -> Sum/2
  MinMax/1 -> acc/1
  Sum/1 -> MinMax/1
  Constant3/1 -> Product1/2
  Constant2/1 -> Product1/1
  Constant1/1 -> MinMax/3
  Product1/1 -> MinMax/2
  brake/1 -> Gain1/1
  throttle/1 -> Gain2/1

== system OptimizationCar/CWSsystem/target/vehicleDynamics/car ==
  brake : Inport
  throttle : Inport  Port=2
  Gain : Gain  Gain=5
  Integrator : Integrator  InitialCondition=targetPosition
  Integrator1 : Integrator  InitialCondition=targetVelocity  LimitOutput=on  LowerSaturationLimit=0
  Sum : Sum  Inputs=|+-
  vehiclePosition : Outport
      settings: AttributesFormatString=signal
  vehicleSpeed : Outport  Port=2
      settings: AttributesFormatString=signal
  wires:
  Integrator/1 -> vehiclePosition/1
  Integrator1/1 -> vehicleSpeed/1, Integrator/1
  Gain/1 -> Integrator1/1
  Sum/1 -> Gain/1
  throttle/1 -> Sum/1
  brake/1 -> Sum/2

== system OptimizationCar/CWSsystem/target/vehicleDynamics/truck ==
  brake : Inport
  throttle : Inport  Port=2
  Gain : Gain  Gain=5
  Integrator : Integrator  InitialCondition=targetPosition
  Integrator1 : Integrator  InitialCondition=targetVelocity  LimitOutput=on  LowerSaturationLimit=0
  Sum : Sum  Inputs=|+-
  vehiclePosition : Outport
      settings: AttributesFormatString=signal
  vehicleSpeed : Outport  Port=2
      settings: AttributesFormatString=signal
  wires:
  brake/1 -> Sum/2
  throttle/1 -> Sum/1
  Sum/1 -> Gain/1
  Gain/1 -> Integrator1/1
  Integrator1/1 -> Integrator/1, vehicleSpeed/1
  Integrator/1 -> vehiclePosition/1

== system OptimizationCar/Constraint/Constraint_1/universally/from ==
  instTrue : Inport
  Constant1 : Constant  Value=0  OutDataTypeStr=uint8
      settings: AttributesFormatString=%<Description>
  Data Type Conversion : DataTypeConversion  OutDataTypeStr=uint8
  Memory : Memory
  Relational Operator2 : RelationalOperator  Operator=>  OutDataTypeStr=boolean  RndMeth=Nearest
  Sum1 : Sum  Inputs=|++
  avoidOverflow : Subsystem
  qualifierTrue : Outport
  wires:
  Memory/1 -> avoidOverflow/1(In)
  Sum1/1 -> Memory/1, Relational Operator2/1
  Constant1/1 -> Relational Operator2/2
  instTrue/1 -> Data Type Conversion/1
  Relational Operator2/1 -> qualifierTrue/1
  Data Type Conversion/1 -> Sum1/1
  avoidOverflow/1(Out) -> Sum1/2

== system OptimizationCar/Constraint/Constraint_1_cond/betweenOC/after ==
  instTrue : Inport
  Constant1 : Constant  Value=0  OutDataTypeStr=uint8
      settings: AttributesFormatString=%<Description>
  Data Type Conversion : DataTypeConversion  OutDataTypeStr=uint8
  Memory : Memory
  Relational Operator2 : RelationalOperator  Operator=>  OutDataTypeStr=boolean  RndMeth=Nearest
  Sum1 : Sum  Inputs=|++
  avoidOverflow : Subsystem
  qualifierTrue : Outport
  wires:
  Memory/1 -> Relational Operator2/1, avoidOverflow/1(In)
  Sum1/1 -> Memory/1
  Constant1/1 -> Relational Operator2/2
  instTrue/1 -> Data Type Conversion/1
  Relational Operator2/1 -> qualifierTrue/1
  Data Type Conversion/1 -> Sum1/1
  avoidOverflow/1(Out) -> Sum1/2

== system OptimizationCar/Constraint/Constraint_1_cond/betweenOC/until ==
  instTrue : Inport
  Constant1 : Constant  OutDataTypeStr=uint8
      settings: AttributesFormatString=%<Description>
  Data Type Conversion : DataTypeConversion  OutDataTypeStr=uint8
  Memory : Memory
  Relational Operator2 : RelationalOperator  Operator=<  OutDataTypeStr=boolean  RndMeth=Nearest
  Sum1 : Sum  Inputs=|++
  avoidOverflow : Subsystem
  qualifierTrue : Outport
  wires:
  Memory/1 -> Relational Operator2/1, avoidOverflow/1(In)
  Sum1/1 -> Memory/1
  Data Type Conversion/1 -> Sum1/1
  Relational Operator2/1 -> qualifierTrue/1
  Constant1/1 -> Relational Operator2/2
  instTrue/1 -> Data Type Conversion/1
  avoidOverflow/1(Out) -> Sum1/2

== system OptimizationCar/Constraint/Constraint_1_cond/existsAndStay/Triggered Subsystem ==
  Trigger : TriggerPort  TriggerType=falling  VariantControl=Variant
  Constant : Constant
  Out1 : Outport  InitialOutput=0
  wires:
  Constant/1 -> Out1/1

== system OptimizationCar/Constraint/Constraint_1_cond/existsAndStay/last ==
  instTrue : Inport
  Enable : EnablePort
  TRUE : Outport  InitialOutput=1
  wires:
  instTrue/1 -> TRUE/1

== system OptimizationCar/Constraint/Constraint_1_cond/existsAndStay/universally ==
  instTrue : Inport
  Enable : EnablePort
  Logical Operator1 : Logic  Operator=NOT  AllPortsSameDT=off  OutDataTypeStr=boolean
  from : Subsystem  TreatAsAtomicUnit=on
  FAULT : Outport  InitialOutput=0
  wires:
  from/1(qualifierTrue) -> FAULT/1
  instTrue/1 -> Logical Operator1/1
  Logical Operator1/1 -> from/1(instTrue)

== system OptimizationCar/Highlevel/Highlevel_1/universally/from ==
  instTrue : Inport
  Constant1 : Constant  Value=0  OutDataTypeStr=uint8
      settings: AttributesFormatString=%<Description>
  Data Type Conversion : DataTypeConversion  OutDataTypeStr=uint8
  Memory : Memory
  Relational Operator2 : RelationalOperator  Operator=>  OutDataTypeStr=boolean  RndMeth=Nearest
  Sum1 : Sum  Inputs=|++
  avoidOverflow : Subsystem
  qualifierTrue : Outport
  wires:
  Memory/1 -> avoidOverflow/1(In)
  Sum1/1 -> Memory/1, Relational Operator2/1
  Constant1/1 -> Relational Operator2/2
  instTrue/1 -> Data Type Conversion/1
  Relational Operator2/1 -> qualifierTrue/1
  Data Type Conversion/1 -> Sum1/1
  avoidOverflow/1(Out) -> Sum1/2

== system OptimizationCar/Highlevel/Highlevel_10/universally/from ==
  instTrue : Inport
  Constant1 : Constant  Value=0  OutDataTypeStr=uint8
      settings: AttributesFormatString=%<Description>
  Data Type Conversion : DataTypeConversion  OutDataTypeStr=uint8
  Memory : Memory
  Relational Operator2 : RelationalOperator  Operator=>  OutDataTypeStr=boolean  RndMeth=Nearest
  Sum1 : Sum  Inputs=|++
  avoidOverflow : Subsystem
  qualifierTrue : Outport
  wires:
  Memory/1 -> avoidOverflow/1(In)
  Sum1/1 -> Memory/1, Relational Operator2/1
  Constant1/1 -> Relational Operator2/2
  instTrue/1 -> Data Type Conversion/1
  Relational Operator2/1 -> qualifierTrue/1
  Data Type Conversion/1 -> Sum1/1
  avoidOverflow/1(Out) -> Sum1/2

== system OptimizationCar/Highlevel/Highlevel_12/universally/from ==
  instTrue : Inport
  Constant1 : Constant  Value=0  OutDataTypeStr=uint8
      settings: AttributesFormatString=%<Description>
  Data Type Conversion : DataTypeConversion  OutDataTypeStr=uint8
  Memory : Memory
  Relational Operator2 : RelationalOperator  Operator=>  OutDataTypeStr=boolean  RndMeth=Nearest
  Sum1 : Sum  Inputs=|++
  avoidOverflow : Subsystem
  qualifierTrue : Outport
  wires:
  Memory/1 -> avoidOverflow/1(In)
  Sum1/1 -> Memory/1, Relational Operator2/1
  Constant1/1 -> Relational Operator2/2
  instTrue/1 -> Data Type Conversion/1
  Relational Operator2/1 -> qualifierTrue/1
  Data Type Conversion/1 -> Sum1/1
  avoidOverflow/1(Out) -> Sum1/2

== system OptimizationCar/Highlevel/Highlevel_13/universally/from ==
  instTrue : Inport
  Constant1 : Constant  Value=0  OutDataTypeStr=uint8
      settings: AttributesFormatString=%<Description>
  Data Type Conversion : DataTypeConversion  OutDataTypeStr=uint8
  Memory : Memory
  Relational Operator2 : RelationalOperator  Operator=>  OutDataTypeStr=boolean  RndMeth=Nearest
  Sum1 : Sum  Inputs=|++
  avoidOverflow : Subsystem
  qualifierTrue : Outport
  wires:
  Memory/1 -> avoidOverflow/1(In)
  Sum1/1 -> Memory/1, Relational Operator2/1
  Constant1/1 -> Relational Operator2/2
  instTrue/1 -> Data Type Conversion/1
  Relational Operator2/1 -> qualifierTrue/1
  Data Type Conversion/1 -> Sum1/1
  avoidOverflow/1(Out) -> Sum1/2

== system OptimizationCar/Highlevel/Highlevel_3/universally/from ==
  instTrue : Inport
  Constant1 : Constant  Value=0  OutDataTypeStr=uint8
      settings: AttributesFormatString=%<Description>
  Data Type Conversion : DataTypeConversion  OutDataTypeStr=uint8
  Memory : Memory
  Relational Operator2 : RelationalOperator  Operator=>  OutDataTypeStr=boolean  RndMeth=Nearest
  Sum1 : Sum  Inputs=|++
  avoidOverflow : Subsystem
  qualifierTrue : Outport
  wires:
  Memory/1 -> avoidOverflow/1(In)
  Sum1/1 -> Memory/1, Relational Operator2/1
  Constant1/1 -> Relational Operator2/2
  instTrue/1 -> Data Type Conversion/1
  Relational Operator2/1 -> qualifierTrue/1
  Data Type Conversion/1 -> Sum1/1
  avoidOverflow/1(Out) -> Sum1/2

== system OptimizationCar/Highlevel/Highlevel_6/universally/from ==
  instTrue : Inport
  Constant1 : Constant  Value=0  OutDataTypeStr=uint8
      settings: AttributesFormatString=%<Description>
  Data Type Conversion : DataTypeConversion  OutDataTypeStr=uint8
  Memory : Memory
  Relational Operator2 : RelationalOperator  Operator=>  OutDataTypeStr=boolean  RndMeth=Nearest
  Sum1 : Sum  Inputs=|++
  avoidOverflow : Subsystem
  qualifierTrue : Outport
  wires:
  Memory/1 -> avoidOverflow/1(In)
  Sum1/1 -> Memory/1, Relational Operator2/1
  Constant1/1 -> Relational Operator2/2
  instTrue/1 -> Data Type Conversion/1
  Relational Operator2/1 -> qualifierTrue/1
  Data Type Conversion/1 -> Sum1/1
  avoidOverflow/1(Out) -> Sum1/2

== system OptimizationCar/Highlevel/Highlevel_7/universally/from ==
  instTrue : Inport
  Constant1 : Constant  Value=0  OutDataTypeStr=uint8
      settings: AttributesFormatString=%<Description>
  Data Type Conversion : DataTypeConversion  OutDataTypeStr=uint8
  Memory : Memory
  Relational Operator2 : RelationalOperator  Operator=>  OutDataTypeStr=boolean  RndMeth=Nearest
  Sum1 : Sum  Inputs=|++
  avoidOverflow : Subsystem
  qualifierTrue : Outport
  wires:
  Memory/1 -> avoidOverflow/1(In)
  Sum1/1 -> Memory/1, Relational Operator2/1
  Constant1/1 -> Relational Operator2/2
  instTrue/1 -> Data Type Conversion/1
  Relational Operator2/1 -> qualifierTrue/1
  Data Type Conversion/1 -> Sum1/1
  avoidOverflow/1(Out) -> Sum1/2

== system OptimizationCar/Assert/Assert_1/existsAndStay/universally/from ==
  instTrue : Inport
  Constant1 : Constant  Value=0  OutDataTypeStr=uint8
      settings: AttributesFormatString=%<Description>
  Data Type Conversion : DataTypeConversion  OutDataTypeStr=uint8
  Memory : Memory
  Relational Operator2 : RelationalOperator  Operator=>  OutDataTypeStr=boolean  RndMeth=Nearest
  Sum1 : Sum  Inputs=|++
  avoidOverflow : Subsystem
  qualifierTrue : Outport
  wires:
  avoidOverflow/1(Out) -> Sum1/2
  Data Type Conversion/1 -> Sum1/1
  Relational Operator2/1 -> qualifierTrue/1
  instTrue/1 -> Data Type Conversion/1
  Constant1/1 -> Relational Operator2/2
  Sum1/1 -> Relational Operator2/1, Memory/1
  Memory/1 -> avoidOverflow/1(In)

== system OptimizationCar/Constraint/Constraint_1/universally/from/avoidOverflow ==
  In : Inport
  Constant : Constant  Value=100
  Constant1 : Constant
  Relational Operator : RelationalOperator  Operator=<  OutDataTypeStr=boolean  RndMeth=Nearest
  Switch : Switch  Criteria=u2 > Threshold  Threshold=0.5
  Out : Outport
  wires:
  Switch/1 -> Out/1
  Constant1/1 -> Switch/3
  Constant/1 -> Relational Operator/2
  In/1 -> Relational Operator/1, Switch/1
  Relational Operator/1 -> Switch/2

== system OptimizationCar/Constraint/Constraint_1_cond/betweenOC/after/avoidOverflow ==
  In : Inport
  Constant : Constant  Value=100
  Constant1 : Constant
  Relational Operator : RelationalOperator  Operator=<  OutDataTypeStr=boolean  RndMeth=Nearest
  Switch : Switch  Criteria=u2 > Threshold  Threshold=0.5
  Out : Outport
  wires:
  Switch/1 -> Out/1
  Constant1/1 -> Switch/3
  Constant/1 -> Relational Operator/2
  In/1 -> Relational Operator/1, Switch/1
  Relational Operator/1 -> Switch/2

== system OptimizationCar/Constraint/Constraint_1_cond/betweenOC/until/avoidOverflow ==
  In : Inport
  Constant : Constant  Value=100
  Constant1 : Constant
  Relational Operator : RelationalOperator  Operator=<  OutDataTypeStr=boolean  RndMeth=Nearest
  Switch : Switch  Criteria=u2 > Threshold  Threshold=0.5
  Out : Outport
  wires:
  Switch/1 -> Out/1
  Constant1/1 -> Switch/3
  Constant/1 -> Relational Operator/2
  In/1 -> Relational Operator/1, Switch/1
  Relational Operator/1 -> Switch/2

== system OptimizationCar/Constraint/Constraint_1_cond/existsAndStay/universally/from ==
  instTrue : Inport
  Constant1 : Constant  Value=0  OutDataTypeStr=uint8
      settings: AttributesFormatString=%<Description>
  Data Type Conversion : DataTypeConversion  OutDataTypeStr=uint8
  Memory : Memory
  Relational Operator2 : RelationalOperator  Operator=>  OutDataTypeStr=boolean  RndMeth=Nearest
  Sum1 : Sum  Inputs=|++
  avoidOverflow : Subsystem
  qualifierTrue : Outport
  wires:
  avoidOverflow/1(Out) -> Sum1/2
  Data Type Conversion/1 -> Sum1/1
  Relational Operator2/1 -> qualifierTrue/1
  instTrue/1 -> Data Type Conversion/1
  Constant1/1 -> Relational Operator2/2
  Sum1/1 -> Relational Operator2/1, Memory/1
  Memory/1 -> avoidOverflow/1(In)

== system OptimizationCar/Highlevel/Highlevel_1/universally/from/avoidOverflow ==
  In : Inport
  Constant : Constant  Value=100
  Constant1 : Constant
  Relational Operator : RelationalOperator  Operator=<  OutDataTypeStr=boolean  RndMeth=Nearest
  Switch : Switch  Criteria=u2 > Threshold  Threshold=0.5
  Out : Outport
  wires:
  Switch/1 -> Out/1
  Constant1/1 -> Switch/3
  Constant/1 -> Relational Operator/2
  In/1 -> Relational Operator/1, Switch/1
  Relational Operator/1 -> Switch/2

== system OptimizationCar/Highlevel/Highlevel_10/universally/from/avoidOverflow ==
  In : Inport
  Constant : Constant  Value=100
  Constant1 : Constant
  Relational Operator : RelationalOperator  Operator=<  OutDataTypeStr=boolean  RndMeth=Nearest
  Switch : Switch  Criteria=u2 > Threshold  Threshold=0.5
  Out : Outport
  wires:
  Switch/1 -> Out/1
  Constant1/1 -> Switch/3
  Constant/1 -> Relational Operator/2
  In/1 -> Relational Operator/1, Switch/1
  Relational Operator/1 -> Switch/2

== system OptimizationCar/Highlevel/Highlevel_12/universally/from/avoidOverflow ==
  In : Inport
  Constant : Constant  Value=100
  Constant1 : Constant
  Relational Operator : RelationalOperator  Operator=<  OutDataTypeStr=boolean  RndMeth=Nearest
  Switch : Switch  Criteria=u2 > Threshold  Threshold=0.5
  Out : Outport
  wires:
  Switch/1 -> Out/1
  Constant1/1 -> Switch/3
  Constant/1 -> Relational Operator/2
  In/1 -> Relational Operator/1, Switch/1
  Relational Operator/1 -> Switch/2

== system OptimizationCar/Highlevel/Highlevel_13/universally/from/avoidOverflow ==
  In : Inport
  Constant : Constant  Value=100
  Constant1 : Constant
  Relational Operator : RelationalOperator  Operator=<  OutDataTypeStr=boolean  RndMeth=Nearest
  Switch : Switch  Criteria=u2 > Threshold  Threshold=0.5
  Out : Outport
  wires:
  Switch/1 -> Out/1
  Constant1/1 -> Switch/3
  Constant/1 -> Relational Operator/2
  In/1 -> Relational Operator/1, Switch/1
  Relational Operator/1 -> Switch/2

== system OptimizationCar/Highlevel/Highlevel_3/universally/from/avoidOverflow ==
  In : Inport
  Constant : Constant  Value=100
  Constant1 : Constant
  Relational Operator : RelationalOperator  Operator=<  OutDataTypeStr=boolean  RndMeth=Nearest
  Switch : Switch  Criteria=u2 > Threshold  Threshold=0.5
  Out : Outport
  wires:
  Switch/1 -> Out/1
  Constant1/1 -> Switch/3
  Constant/1 -> Relational Operator/2
  In/1 -> Relational Operator/1, Switch/1
  Relational Operator/1 -> Switch/2
